simulink model "New_FOC_old0x2820x29"  (R2024b)
settings: Solver=FixedStepAuto  StartTime=0.0  StopTime=2.5  FixedStep=1e-6  MaxStep=1e-3
values from neighbouring files (symbols this model uses):
  Ki_d = (wn_d^2) / b_d    (= 228532.608696)    [FOC_Code.m]
  Ki_q = (wn_q^2) / b_q    (= 228532.608696)    [FOC_Code.m]
  Ki_s = (wn_s^2) / b_s    [FOC_Code.m]
  Kp_d = (2*zeta*wn_d - a_d) / b_d    (= 62.35)    [FOC_Code.m]
  Kp_q = (2*zeta*wn_q - a_q) / b_q    (= 62.35)    [FOC_Code.m]
  Kp_s = (2*zeta*wn_s - a_s) / b_s    [FOC_Code.m]
  lambda = 0.0884669    [FOC_Code.m]
  Ld = 5.75e-3    (= 0.00575)    [FOC_Code.m]
  Lq = 5.75e-3    (= 0.00575)    [FOC_Code.m]
  ma = 0.95    [FOC_Code.m]
  p = 3    [FOC_Code.m]
  T_max = 3.81    [FOC_Code.m]
  T_period = 1/fs    (= 0.0001)    [FOC_Code.m]
  Vdc = 311    [FOC_Code.m]
libraries: spsIGBTDiodeLib x12, simulink x9, spsCurrentMeasurementLib x6, spsVoltageMeasurementLib x6, spsStairGeneratorLib x3, spsDCVoltageSourceLib x2, spsPermanentMagnetSynchronousMachineLib x2, spsTriangleGeneratorLib x1, spspowerguiLib x1, sps_lib x1
settings Model: Creator=FSOS  LastModifiedBy=Habiba
settings SolverCC: ZeroCrossAlgorithm=Adaptive  AlgebraicLoopSolver=TrustRegion
settings DebuggingCC: IgnoredZcDiagnostic=none  ArithmeticOperatorsInVariantConditions=warning
settings SFSimCC: CustomCodeUndefinedFunction=UseInterfaceOnly
settings RTWCC: GPUComputeCapability=3.5

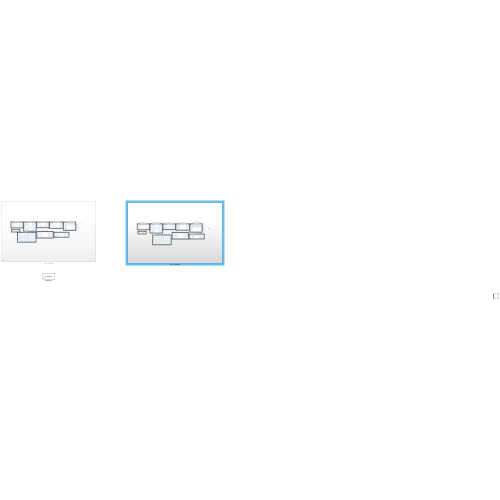
[thumbnail: Simulink's stored preview of the top-level diagram]
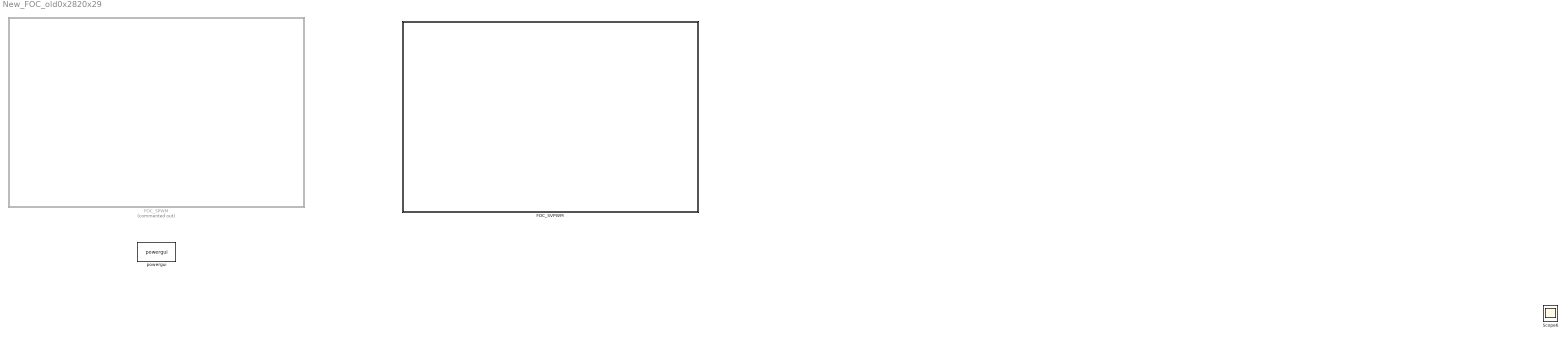
== system New_FOC_old0x2820x29 ==
  FOC_SPWM : Subsystem  Commented=on
  FOC_SVPWM : Subsystem
  Scope6 : Scope  NumInputPorts=3
  powergui : sps_lib/powergui  Priority=1  SimulationMode=Continuous  SampleTime=50e-6  frequency=60  Iterations=50  frequencyindice=0  Pbase=100e6  ErrMax=1e-4  UnitsV=kV  UnitsW=MW  buscounter=0  FunctionMessages=off  echomessages=off  EnableUseOfTLC=off  CurrentSourceSwitches=off  DisableSnubberDevices=off  DisableRonSwitches=off  DisableVfSwitches=off  DisplayEquations=off  AutomaticDiscreteSolvers=off  SolverType=Tustin/Backward Euler (TBE)  Interpol=off  ExternalGateDelay=off  methode=off  Ts=100  x0status=blocks  SPID=on  SwTol=0  HookPort=off  NonlinearTolerance=1e-4  nMaxIteration=100  ContinueOnMaxIteration=off  RestoreLinks=warning  ResistiveCurrentMeasurement=off  Frange=[0:2:500]  Ylog=off  Xlog=on  ShowGrid=off  save=off  variable=ZData  structure=0  ZoomFFT=off  StartTime=0.0  cycles=1  DisplayStyle=1  fundamental=60  FreqAxis=off  MaxFrequency=1000  frequencyindicesteady=1  RmsSteady=1  display=off

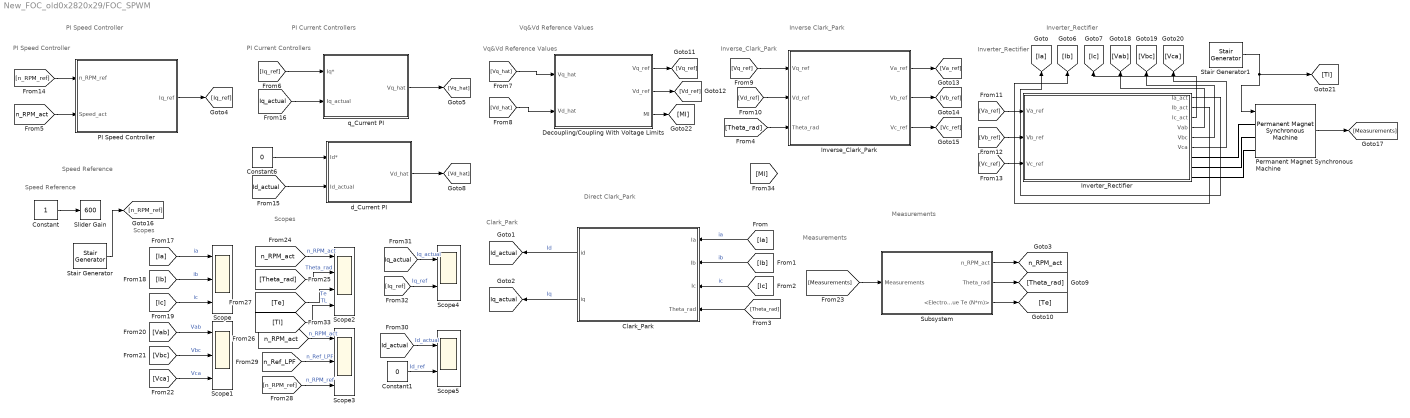
== system New_FOC_old0x2820x29/FOC_SPWM ==
  note: Scopes
  note: Measurements
  note: Speed Reference
  note: Inverter_Rectifier
  note: Clark_Park
  note: Inverse_Clark_Park
  note: Vq&Vd Reference Values
  note: PI Current Controllers
  note: PI Speed Controller
  note: PI Speed Controller
  note: PI Current Controllers
  note: Vq&Vd Reference Values
  note: Inverse Clark_Park
  note: Direct Clark_Park
  note: Inverter_Rectifier
  note: Speed Reference
  note: Measurements
  note: Scopes
  Clark_Park : Subsystem
  Constant : Constant
  Constant1 : Constant  Value=0
  Constant6 : Constant  Value=0
  Decoupling/Coupling With Voltage Limits : Subsystem
  Inverse_Clark_Park : Subsystem
  Inverter_Rectifier : Subsystem
  PI Speed Controller : Subsystem
  Permanent Magnet Synchronous Machine : spsPermanentMagnetSynchronousMachineLib/Permanent Magnet Synchronous Machine  NbPhases=3  FluxDistribution=Sinusoidal  RotorType=Round  MechanicalLoad=Torque Tm  PresetModel="01:  0.8 Nm 300 Vdc 3000 RPM - 0.8 Nm"  ShowDetailedParameters=on  MeasurementBus=off  Resistance=18.7  Inductance=8.5e-3  dqInductances=[0.006047 0.006683]  La=0.02682  MachineConstant=Flux linkage established by magnets (V.s)  Flux=0.1716  VoltageCst=62.2496  TorqueCst=0.5148  Flat=120  Mechanical=[2.26e-05 1.349e-05 2 0]  PolePairs=2  InitialConditions=[0,0, 0,0]  InitialConditions5ph=[0 0 0 0 0 0]  RefAngle=Aligned with phase A axis (original Park)  IterativeDiscreteModel=Trapezoidal non iterative  TsBlock=-1  TsPowergui=0
  Scope : Scope  NumInputPorts=3
  Scope1 : Scope  NumInputPorts=3
  Scope2 : Scope  NumInputPorts=4
  Scope3 : Scope  NumInputPorts=3
  Scope4 : Scope  NumInputPorts=2
  Scope5 : Scope  NumInputPorts=2
  Slider Gain : simulink/Math Operations/Slider Gain  gain=600  low=0  high=3000
  Stair Generator : spsStairGeneratorLib/Stair Generator  t=[0 .15 .3 .45 .7 .85 1 1.15 1.3]  e=[200 2000 500 3000 0 -1000 -2500 0 2500]  Ts=1e-5
  Stair Generator1 : spsStairGeneratorLib/Stair Generator  t=[0 1.3 1.45 1.6 1.75 1.9 2]  e=[0 1.5 2 2.8 2.5 .8 2.2]  Ts=0
  Subsystem : Subsystem
  d_Current PI : Subsystem
  q_Current PI : Subsystem
  tag scope: Id_actual=global, Iq_actual=global, n_RPM_act=global
  wires:
  Subsystem/2(Theta_rad) -> [Theta_rad]
  Constant6/1 -> d_Current PI/1(Id*)
  [Vd_ref] -> Inverse_Clark_Park/2(Vd_ref)
  [Vq_ref] -> Inverse_Clark_Park/1(Vq_ref)
  [n_RPM_ref] -> PI Speed Controller/1(n_RPM_ref)
  [Iq_actual] -> Scope4/1  "Iq_actual"
  [Id_actual] -> d_Current PI/2(Id_actual)
  Inverter_Rectifier/2(Ib_act) -> [Ib]
  [Ic] -> Clark_Park/3(Ic)  "ic"
  Inverse_Clark_Park/2(Vb_ref) -> [Vb_ref]
  Clark_Park/2(iq) -> [Iq_actual]  "Iq"
  [n_RPM_act] -> PI Speed Controller/2(Speed_act)
  [Ia] -> Scope/1  "ia"
  Clark_Park/1(id) -> [Id_actual]  "Id"
  [Iq_actual] -> q_Current PI/2(Iq_actual)
  [Iq_ref] -> Scope4/2  "Iq_ref"
  Decoupling/Coupling With Voltage Limits/2(Vd_ref) -> [Vd_ref]
  [Ib] -> Scope/2  "ib"
  Constant/1 -> Slider Gain/1
  [Ib] -> Clark_Park/2(Ib)  "ib"
  Inverter_Rectifier/5(Vbc) -> [Vbc]
  [Theta_rad] -> Inverse_Clark_Park/3(Theta_rad)
  [Id_actual] -> Scope5/1  "Id_actual"
  [Ia] -> Clark_Park/1(Ia)  "ia"
  [Theta_rad] -> Clark_Park/4(Theta_rad)
  [Measurements] -> Subsystem/1(Measurements)
  [Vq_hat] -> Decoupling/Coupling With Voltage Limits/1(Vq_hat)
  Decoupling/Coupling With Voltage Limits/1(Vq_ref) -> [Vq_ref]
  PI Speed Controller/1(Iq_ref) -> [Iq_ref]
  [Vca] -> Scope1/3  "Vca"
  d_Current PI/1(Vd_hat) -> [Vd_hat]
  [Vd_hat] -> Decoupling/Coupling With Voltage Limits/2(Vd_hat)
  [Va_ref] -> Inverter_Rectifier/1(Va_ref)
  Constant1/1 -> Scope5/2  "Id_ref"
  [Vc_ref] -> Inverter_Rectifier/3(Vc_ref)
  [n_RPM_act] -> Scope2/1  "n_RPM_act"
  Inverse_Clark_Park/3(Vc_ref) -> [Vc_ref]
  Inverter_Rectifier/6(Vca) -> [Vca]
  [Iq_ref] -> q_Current PI/1(Iq*)
  [Vab] -> Scope1/1  "Vab"
  q_Current PI/1(Vq_hat) -> [Vq_hat]
  Inverter_Rectifier/1(Ia_act) -> [Ia]
  [n_RPM_act] -> Scope3/1  "n_RPM_act"
  [Vb_ref] -> Inverter_Rectifier/2(Vb_ref)
  Subsystem/1(n_RPM_act) -> [n_RPM_act]
  [Theta_rad] -> Scope2/2  "Theta_rad"
  Inverter_Rectifier/4(Vab) -> [Vab]
  Inverter_Rectifier/3(Ic_act) -> [Ic]
  Inverse_Clark_Park/1(Va_ref) -> [Va_ref]
  [Te] -> Scope2/3  "Te"
  Subsystem/3(<Electromagnetic torque Te (N*m)>) -> [Te]
  [Ic] -> Scope/3  "ic"
  [Vbc] -> Scope1/2  "Vbc"
  Permanent Magnet Synchronous Machine/1 -> [Measurements]
  Stair Generator1/1 -> Permanent Magnet Synchronous Machine/1, [Tl]
  [Tl] -> Scope2/4  "TL"
  [n_Ref_LPF] -> Scope3/2  "n_Ref_LPF"
  [n_RPM_ref] -> Scope3/3  "n_RPM_ref"
  Decoupling/Coupling With Voltage Limits/3(MI) -> [MI]
  Stair Generator/1 -> [n_RPM_ref]
  connections:
  Permanent Magnet Synchronous Machine/LConn2 -- Inverter_Rectifier/RConn2
  Permanent Magnet Synchronous Machine/LConn1 -- Inverter_Rectifier/RConn1
  Permanent Magnet Synchronous Machine/LConn3 -- Inverter_Rectifier/RConn3

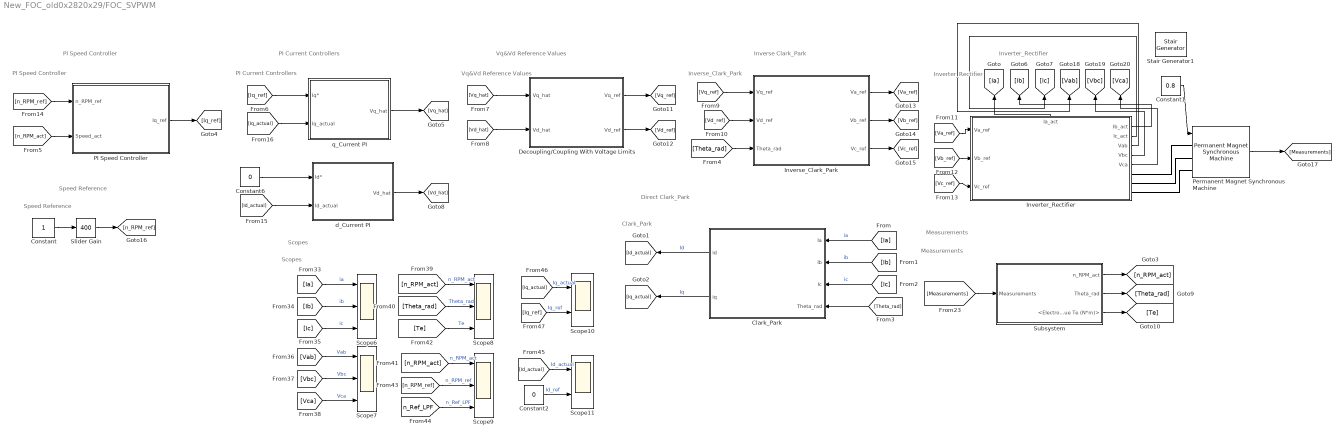
== system New_FOC_old0x2820x29/FOC_SVPWM ==
  note: Measurements
  note: Speed Reference
  note: Inverter_Rectifier
  note: Direct Clark_Park
  note: Inverse Clark_Park
  note: Vq&Vd Reference Values
  note: PI Current Controllers
  note: PI Speed Controller
  note: PI Speed Controller
  note: PI Current Controllers
  note: Vq&Vd Reference Values
  note: Inverse_Clark_Park
  note: Clark_Park
  note: Inverter_Rectifier
  note: Speed Reference
  note: Measurements
  note: Scopes
  note: Scopes
  Clark_Park : Subsystem
  Constant : Constant
  Constant1 : Constant  Value=0.8
  Constant2 : Constant  Value=0
  Constant6 : Constant  Value=0
  Decoupling/Coupling With Voltage Limits : Subsystem
  Inverse_Clark_Park : Subsystem
  Inverter_Rectifier : Subsystem
      settings: PortSchema="{\"entries\":[{\"content\":{\"sides\":[{\"content\":{\"connectorIds\":[\"In1\",\"In2\",\"In3\"]},\"type\":\"ConnectorPlacement.EquallySpacedRectSide\",\"uuid\":\"7414f413-f740-4713-9a5b-35e41764df99\"},{\"content\":{\"connectorIds\":[\"Out1\",\"Out2\",\"Out3\",\"Out4\",\"Out5\",\"RConn1\",\"RConn2\",\"RConn3\"],\"side\":\"RIGHT\"},\"type\":\"ConnectorPlacement.EquallySpacedRectSide\",\"uuid\":\"0ae7f1d1-4f19-4170-a25f-9376873eedc4\"},{\"content\":{\"connectorIds\":[\"Out6\"],\"side\":\"TOP\"},\"type\":\"ConnectorPlacement.EquallySpacedRectSide\",\"uuid\":\"dcf59177-a21c-40cb-b25d-eb83961f197b\"}]},\"type\":\"ConnectorPlacement.EquallySpacedConnector\",\"uuid\":\"0cdaba68-969f-44b0-8b53-9ca11596f6f2\"}],\"packageUris\":[\"http://schema.mathworks.com/mf0/Connector/R2020b\"],\"version\":\"1.0\"}"
  PI Speed Controller : Subsystem
  Permanent Magnet Synchronous Machine : spsPermanentMagnetSynchronousMachineLib/Permanent Magnet Synchronous Machine  NbPhases=3  FluxDistribution=Sinusoidal  RotorType=Round  MechanicalLoad=Torque Tm  PresetModel=No  ShowDetailedParameters=on  MeasurementBus=off  Resistance=2.9  Inductance=8.5e-3  dqInductances=[0.006047 0.006683]  La=5.75e-3  MachineConstant=Flux linkage established by magnets (V.s)  Flux=0.0884669  VoltageCst=48.1384  TorqueCst=0.3981  Flat=120  Mechanical=[0.405e-4 0.0314 3 0]  PolePairs=2  InitialConditions=[0,0, 0,0]  InitialConditions5ph=[0 0 0 0 0 0]  RefAngle=Aligned with phase A axis (original Park)  IterativeDiscreteModel=Trapezoidal non iterative  TsBlock=-1  TsPowergui=0
  Scope10 : Scope  NumInputPorts=2
  Scope11 : Scope  NumInputPorts=2
  Scope{6..9} (4 alike) : Scope  NumInputPorts=3
  Slider Gain : simulink/Math Operations/Slider Gain  gain=400  low=0  high=3000
  Stair Generator1 : spsStairGeneratorLib/Stair Generator  t=[0 1.3 1.45 1.6 1.75 1.9 2]  e=[0 1.5 2 2.8 2.5 .8 2.2]  Ts=0
  Subsystem : Subsystem
  d_Current PI : Subsystem
  q_Current PI : Subsystem
  wires:
  Permanent Magnet Synchronous Machine/1 -> [Measurements]
  Subsystem/3(<Electromagnetic torque Te (N*m)>) -> [Te]
  Inverse_Clark_Park/1(Va_ref) -> [Va_ref]
  Inverter_Rectifier/2(Ic_act) -> [Ic]
  Inverter_Rectifier/3(Vab) -> [Vab]
  Subsystem/1(n_RPM_act) -> [n_RPM_act]
  [Vb_ref] -> Inverter_Rectifier/2(Vb_ref)
  Inverter_Rectifier/6(Ia_act) -> [Ia]
  q_Current PI/1(Vq_hat) -> [Vq_hat]
  [Iq_ref] -> q_Current PI/1(Iq*)
  Inverter_Rectifier/5(Vca) -> [Vca]
  Inverse_Clark_Park/3(Vc_ref) -> [Vc_ref]
  [Vc_ref] -> Inverter_Rectifier/3(Vc_ref)
  [Va_ref] -> Inverter_Rectifier/1(Va_ref)
  [Vd_hat] -> Decoupling/Coupling With Voltage Limits/2(Vd_hat)
  d_Current PI/1(Vd_hat) -> [Vd_hat]
  PI Speed Controller/1(Iq_ref) -> [Iq_ref]
  Decoupling/Coupling With Voltage Limits/1(Vq_ref) -> [Vq_ref]
  [Vq_hat] -> Decoupling/Coupling With Voltage Limits/1(Vq_hat)
  [Measurements] -> Subsystem/1(Measurements)
  [Theta_rad] -> Clark_Park/4(Theta_rad)
  [Ia] -> Clark_Park/1(Ia)  "ia"
  [Theta_rad] -> Inverse_Clark_Park/3(Theta_rad)
  Inverter_Rectifier/4(Vbc) -> [Vbc]
  [Ib] -> Clark_Park/2(Ib)  "ib"
  Constant/1 -> Slider Gain/1
  Decoupling/Coupling With Voltage Limits/2(Vd_ref) -> [Vd_ref]
  [Iq_actual] -> q_Current PI/2(Iq_actual)
  Clark_Park/1(id) -> [Id_actual]  "Id"
  [n_RPM_act] -> PI Speed Controller/2(Speed_act)
  Clark_Park/2(iq) -> [Iq_actual]  "Iq"
  Inverse_Clark_Park/2(Vb_ref) -> [Vb_ref]
  [Ic] -> Clark_Park/3(Ic)  "ic"
  Inverter_Rectifier/1(Ib_act) -> [Ib]
  [Id_actual] -> d_Current PI/2(Id_actual)
  [n_RPM_ref] -> PI Speed Controller/1(n_RPM_ref)
  [Vq_ref] -> Inverse_Clark_Park/1(Vq_ref)
  [Vd_ref] -> Inverse_Clark_Park/2(Vd_ref)
  Constant6/1 -> d_Current PI/1(Id*)
  Subsystem/2(Theta_rad) -> [Theta_rad]
  [n_RPM_act] -> Scope9/1  "n_RPM_act"
  [n_RPM_act] -> Scope8/1  "n_RPM_act"
  [Theta_rad] -> Scope8/2  "Theta_rad"
  [Vca] -> Scope7/3  "Vca"
  [Ia] -> Scope6/1  "ia"
  [n_Ref_LPF] -> Scope9/3  "n_Ref_LPF"
  [Id_actual] -> Scope11/1  "Id_actual"
  Constant2/1 -> Scope11/2  "Id_ref"
  [Iq_actual] -> Scope10/1  "Iq_actual"
  [Vbc] -> Scope7/2  "Vbc"
  [Te] -> Scope8/3  "Te"
  [Iq_ref] -> Scope10/2  "Iq_ref"
  [Vab] -> Scope7/1  "Vab"
  [Ic] -> Scope6/3  "ic"
  [n_RPM_ref] -> Scope9/2  "n_RPM_ref"
  [Ib] -> Scope6/2  "ib"
  Constant1/1 -> Permanent Magnet Synchronous Machine/1
  Slider Gain/1 -> [n_RPM_ref]
  connections:
  Permanent Magnet Synchronous Machine/LConn3 -- Inverter_Rectifier/RConn3
  Permanent Magnet Synchronous Machine/LConn1 -- Inverter_Rectifier/RConn1
  Permanent Magnet Synchronous Machine/LConn2 -- Inverter_Rectifier/RConn2

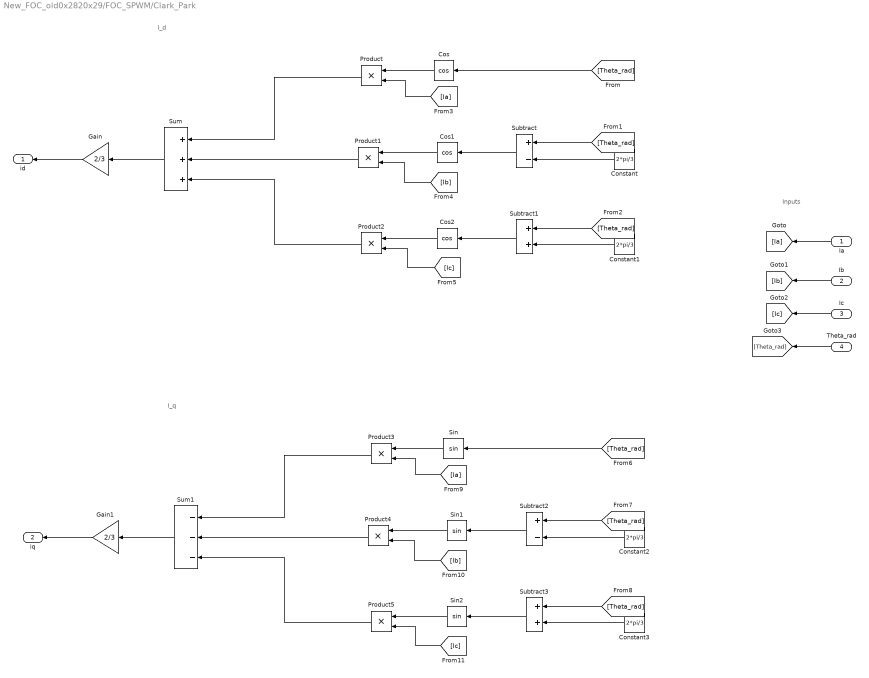
== system New_FOC_old0x2820x29/FOC_SPWM/Clark_Park ==
  note: Inputs
  note: I_d
  note: I_q
  Ia : Inport
  Ib : Inport  Port=2
  Ic : Inport  Port=3
  Theta_rad : Inport  Port=4
  Constant{,1..3} (4 alike) : Constant  Value=2*pi/3
  Cos : Trigonometry  Operator=cos
  Cos1 : Trigonometry  Operator=cos
  Cos2 : Trigonometry  Operator=cos
  Gain : Gain  Gain=2/3
  Gain1 : Gain  Gain=2/3
  Product{,1..5} (6 alike) : Product
  Sin : Trigonometry
  Sin1 : Trigonometry
  Sin2 : Trigonometry
  Subtract : Sum  Inputs=+-
  Subtract1 : Sum
  Subtract2 : Sum  Inputs=+-
  Subtract3 : Sum
  Sum : Sum  Inputs=+++
  Sum1 : Sum  Inputs=---
  id : Outport
  iq : Outport  Port=2
  wires:
  Ia/1 -> [Ia]
  Ib/1 -> [Ib]
  Ic/1 -> [Ic]
  Theta_rad/1 -> [Theta_rad]
  Cos/1 -> Product/1
  Cos1/1 -> Product1/1
  Cos2/1 -> Product2/1
  [Theta_rad] -> Cos/1
  Subtract/1 -> Cos1/1
  [Theta_rad] -> Subtract/1
  Constant/1 -> Subtract/2
  Constant1/1 -> Subtract1/2
  [Theta_rad] -> Subtract1/1
  Subtract1/1 -> Cos2/1
  [Ia] -> Product/2
  [Ib] -> Product1/2
  [Ic] -> Product2/2
  Product1/1 -> Sum/2
  Product/1 -> Sum/1
  Product2/1 -> Sum/3
  Sum/1 -> Gain/1
  Gain/1 -> id/1
  Gain1/1 -> iq/1
  Sum1/1 -> Gain1/1
  Product5/1 -> Sum1/3
  Product3/1 -> Sum1/1
  Product4/1 -> Sum1/2
  [Ic] -> Product5/2
  [Ib] -> Product4/2
  [Ia] -> Product3/2
  Subtract3/1 -> Sin2/1
  [Theta_rad] -> Subtract3/1
  Constant3/1 -> Subtract3/2
  Constant2/1 -> Subtract2/2
  [Theta_rad] -> Subtract2/1
  Subtract2/1 -> Sin1/1
  [Theta_rad] -> Sin/1
  Sin2/1 -> Product5/1
  Sin1/1 -> Product4/1
  Sin/1 -> Product3/1

== system New_FOC_old0x2820x29/FOC_SPWM/Decoupling//Coupling With Voltage Limits ==
  note: MI_Calculations
  Vq_hat : Inport
  Vd_hat : Inport  Port=2
  Decoupling/Coupling : Subsystem
  MI_Calculations : Subsystem
  Voltage Limited : Subsystem
  Vq_ref : Outport
  Vd_ref : Outport  Port=2
  MI : Outport  Port=3
  wires:
  Decoupling/Coupling/1(Vq) -> Voltage Limited/1(Vq)
  Decoupling/Coupling/2(Vd) -> Voltage Limited/2(Vd)
  Vq_hat/1 -> Decoupling/Coupling/1(Vq_hat)
  Voltage Limited/1(Vq_ref) -> MI_Calculations/1(Vq_ref), Vq_ref/1
  Vd_hat/1 -> Decoupling/Coupling/2(Vd_hat)
  MI_Calculations/1(MI) -> MI/1
  Voltage Limited/2(Vd_ref) -> MI_Calculations/2(Vd_ref), Vd_ref/1

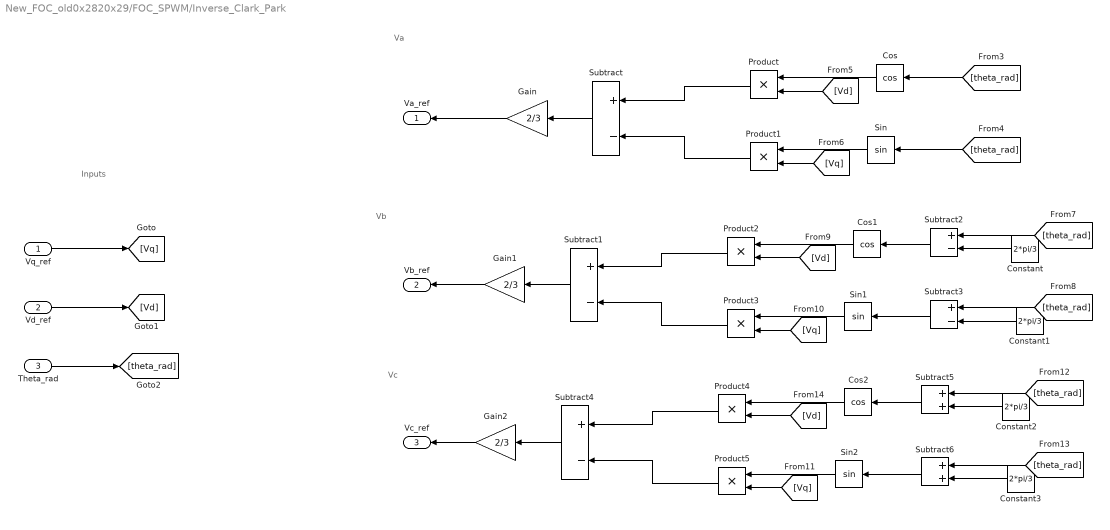
== system New_FOC_old0x2820x29/FOC_SPWM/Inverse_Clark_Park ==
  note: Vc
  note: Vb
  note: Va
  note: Inputs
  Vq_ref : Inport
  Vd_ref : Inport  Port=2
  Theta_rad : Inport  Port=3
  Constant{,1..3} (4 alike) : Constant  Value=2*pi/3
  Cos : Trigonometry  Operator=cos
  Cos1 : Trigonometry  Operator=cos
  Cos2 : Trigonometry  Operator=cos
  Gain : Gain  Gain=2/3
  Gain1 : Gain  Gain=2/3
  Gain2 : Gain  Gain=2/3
  Product{,1..5} (6 alike) : Product
  Sin : Trigonometry
  Sin1 : Trigonometry
  Sin2 : Trigonometry
  Subtract{,1..4} (5 alike) : Sum  Inputs=+-
  Subtract5 : Sum
  Subtract6 : Sum
  Va_ref : Outport
  Vb_ref : Outport  Port=2
  Vc_ref : Outport  Port=3
  wires:
  Vq_ref/1 -> [Vq]
  Vd_ref/1 -> [Vd]
  Theta_rad/1 -> [theta_rad]
  [theta_rad] -> Cos/1
  [theta_rad] -> Sin/1
  Cos/1 -> Product/1
  Sin/1 -> Product1/1
  [Vd] -> Product/2
  [Vq] -> Product1/2
  Product/1 -> Subtract/1
  Product1/1 -> Subtract/2
  Subtract/1 -> Gain/1
  Gain/1 -> Va_ref/1
  Subtract1/1 -> Gain1/1
  Product3/1 -> Subtract1/2
  Product2/1 -> Subtract1/1
  [Vq] -> Product3/2
  [Vd] -> Product2/2
  Sin1/1 -> Product3/1
  Cos1/1 -> Product2/1
  Subtract2/1 -> Cos1/1
  [theta_rad] -> Subtract2/1
  Subtract3/1 -> Sin1/1
  [theta_rad] -> Subtract3/1
  Constant/1 -> Subtract2/2
  Constant1/1 -> Subtract3/2
  Gain1/1 -> Vb_ref/1
  Gain2/1 -> Vc_ref/1
  Constant3/1 -> Subtract6/2
  Constant2/1 -> Subtract5/2
  [theta_rad] -> Subtract6/1
  Subtract6/1 -> Sin2/1
  [theta_rad] -> Subtract5/1
  Subtract5/1 -> Cos2/1
  Cos2/1 -> Product4/1
  Sin2/1 -> Product5/1
  [Vd] -> Product4/2
  [Vq] -> Product5/2
  Product4/1 -> Subtract4/1
  Product5/1 -> Subtract4/2
  Subtract4/1 -> Gain2/1

== system New_FOC_old0x2820x29/FOC_SPWM/Inverter_Rectifier ==
  Va_ref : Inport
  Vb_ref : Inport  Port=2
  Vc_ref : Inport  Port=3
  Current Measurement : spsCurrentMeasurementLib/Current Measurement  PhasorSimulation=off  OutputType=Complex  PSBequivalent=0
  Current Measurement1 : spsCurrentMeasurementLib/Current Measurement  PhasorSimulation=off  OutputType=Complex  PSBequivalent=0
  Current Measurement2 : spsCurrentMeasurementLib/Current Measurement  PhasorSimulation=off  OutputType=Complex  PSBequivalent=0
  Inverter_SPWM : Subsystem
  Voltage Measurement : spsVoltageMeasurementLib/Voltage Measurement  PhasorSimulation=off  OutputType=Complex  PSBequivalent=0
  Voltage Measurement1 : spsVoltageMeasurementLib/Voltage Measurement  PhasorSimulation=off  OutputType=Complex  PSBequivalent=0
  Voltage Measurement2 : spsVoltageMeasurementLib/Voltage Measurement  PhasorSimulation=off  OutputType=Complex  PSBequivalent=0
  Va_act : PMIOPort  Side=Right
  Vb_act : PMIOPort  Port=2  Side=Right
  Vc_act : PMIOPort  Port=3  Side=Right
  Ia_act : Outport
  Ib_act : Outport  Port=2
  Ic_act : Outport  Port=3
  Vab : Outport  Port=4
  Vbc : Outport  Port=5
  Vca : Outport  Port=6
  wires:
  Current Measurement/1 -> Ia_act/1
  Vc_ref/1 -> Inverter_SPWM/3(Vc_ref)
  Current Measurement2/1 -> Ic_act/1
  Current Measurement1/1 -> Ib_act/1
  Vb_ref/1 -> Inverter_SPWM/2(Vb_ref)
  Va_ref/1 -> Inverter_SPWM/1(Va_ref)
  Voltage Measurement/1 -> Vab/1
  Voltage Measurement1/1 -> Vbc/1
  Voltage Measurement2/1 -> Vca/1
  connections:
  Current Measurement/RConn1 -- Va_act/RConn1
  Current Measurement1/RConn1 -- Vb_act/RConn1
  Current Measurement/LConn1 -- Inverter_SPWM/RConn1 -- Voltage Measurement2/LConn2 -- Voltage Measurement/LConn1
  Inverter_SPWM/RConn3 -- Voltage Measurement1/LConn2 -- Current Measurement2/LConn1 -- Voltage Measurement2/LConn1
  Inverter_SPWM/RConn2 -- Voltage Measurement/LConn2 -- Current Measurement1/LConn1 -- Voltage Measurement1/LConn1
  Current Measurement2/RConn1 -- Vc_act/RConn1

== system New_FOC_old0x2820x29/FOC_SPWM/PI Speed Controller ==
  note: في لوك لتحويل للrad/s
  note: Subsystem2
  n_RPM_ref : Inport
  Speed_act : Inport  Port=2
  Abs : Abs  SaturateOnIntegerOverflow=off
  Abs1 : Abs  SaturateOnIntegerOverflow=off
  Compare To Constant : simulink/Logic and Bit Operations/Compare To Constant  relop=<=  const=0.0001  OutDataTypeStr=boolean
  For stop integral in the starting : Relay  OnSwitchValue=100  OffSwitchValue=-100
  Gain : Gain  Gain=Kp_s
  Gain1 : Gain  Gain=Ki_s
  Integrator1 : Integrator
  Iq_Max : Saturate  UpperLimit=T_max*2/(3*p*lambda)  LowerLimit=-(2*T_max) / (3*p*lambda)
  LPF : TransferFcn  Denominator=[1/100 1]
  Product : Product  Inputs=3
  Sum : Sum  Inputs=|+-
  Sum3 : Sum  Inputs=|++
  Sum4 : Sum  Inputs=|-+
  Iq_ref : Outport
  tag scope: n_Ref_LPF=global
  wires:
  Speed_act/1 -> Abs1/1, Sum/2
  Iq_Max/1 -> Iq_ref/1, Sum4/1
  LPF/1 -> [n_Ref_LPF], Sum/1
  Gain1/1 -> Product/2
  Sum3/1 -> Sum4/2, Iq_Max/1
  Gain/1 -> Sum3/1
  Abs1/1 -> For stop integral in the starting/1
  Product/1 -> Integrator1/1
  For stop integral in the starting/1 -> Product/3
  Integrator1/1 -> Sum3/2
  Sum4/1 -> Abs/1
  Abs/1 -> Compare To Constant/1
  Compare To Constant/1 -> Product/1
  n_RPM_ref/1 -> LPF/1
  Sum/1 -> Gain1/1, Gain/1

== system New_FOC_old0x2820x29/FOC_SPWM/Subsystem ==
  Measurements : Inport
  0-2pi : Math  Operator=rem  SignedPower=on
  Bus Selector : BusSelector  OutputSignals=Rotor speed wm (rad/s),Rotor angle thetam (rad),Electromagnetic torque Te (N*m)
  Constant7 : Constant  Value=2*pi
  Gain2 : Gain  Gain=30/pi
  mech to elec1 : Gain  Gain=p
  n_RPM_act : Outport
  Theta_rad : Outport  Port=2
  <Electromagnetic torque Te (N*m)> : Outport  Port=3
  wires:
  Constant7/1 -> 0-2pi/2
  Measurements/1 -> Bus Selector/1
  Gain2/1 -> n_RPM_act/1
  Bus Selector/1 -> Gain2/1  "<Rotor speed wm (rad/s)>"
  Bus Selector/2 -> mech to elec1/1  "<Rotor angle thetam (rad)>"
  Bus Selector/3 -> <Electromagnetic torque Te (N*m)>/1  "<Electromagnetic torque Te (N*m)>"
  0-2pi/1 -> Theta_rad/1
  mech to elec1/1 -> 0-2pi/1

== system New_FOC_old0x2820x29/FOC_SPWM/d_Current PI ==
  Id* : Inport
  Id_actual : Inport  Port=2
  Gain : Gain  Gain=Kp_d
  Gain1 : Gain  Gain=Ki_d
  Integrator : Integrator
  Product : Product
  Sum : Sum  Inputs=|+-
  Sum1 : Sum  Inputs=|++
  Vd_hat : Outport
  wires:
  Sum1/1 -> Vd_hat/1
  Gain1/1 -> Product/1
  Gain/1 -> Sum1/1
  Sum/1 -> Gain/1, Gain1/1
  Id_actual/1 -> Sum/2
  Id*/1 -> Sum/1
  [Stop_d] -> Product/2  "act as anti wind-up"
  Product/1 -> Integrator/1
  Integrator/1 -> Sum1/2

== system New_FOC_old0x2820x29/FOC_SPWM/q_Current PI ==
  Iq* : Inport
  Iq_actual : Inport  Port=2
  Gain : Gain  Gain=Kp_q
  Gain1 : Gain  Gain=Ki_q
  Integrator : Integrator
  Product : Product
  Sum : Sum  Inputs=|+-
  Sum1 : Sum  Inputs=|++
  Vq_hat : Outport
  wires:
  Iq*/1 -> Sum/1
  Iq_actual/1 -> Sum/2
  Sum/1 -> Gain1/1, Gain/1
  Gain/1 -> Sum1/1
  Gain1/1 -> Product/1
  Sum1/1 -> Vq_hat/1
  [Stop_q] -> Product/2  "act as anti wind-up"
  Integrator/1 -> Sum1/2
  Product/1 -> Integrator/1

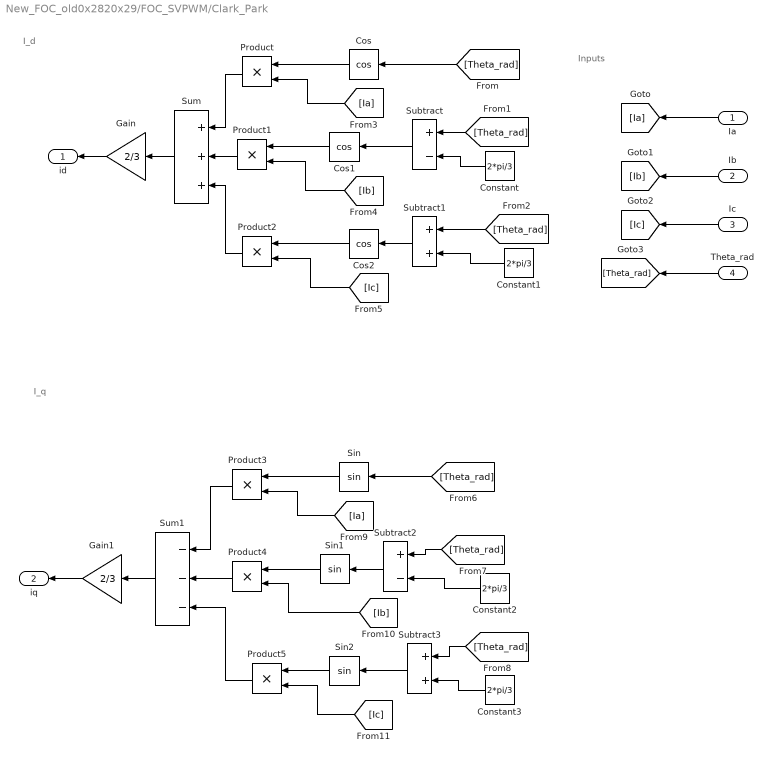
== system New_FOC_old0x2820x29/FOC_SVPWM/Clark_Park ==
  note: I_q
  note: I_d
  note: Inputs
  Ia : Inport
  Ib : Inport  Port=2
  Ic : Inport  Port=3
  Theta_rad : Inport  Port=4
  Constant{,1..3} (4 alike) : Constant  Value=2*pi/3
  Cos : Trigonometry  Operator=cos
  Cos1 : Trigonometry  Operator=cos
  Cos2 : Trigonometry  Operator=cos
  Gain : Gain  Gain=2/3
  Gain1 : Gain  Gain=2/3
  Product{,1..5} (6 alike) : Product
  Sin : Trigonometry
  Sin1 : Trigonometry
  Sin2 : Trigonometry
  Subtract : Sum  Inputs=+-
  Subtract1 : Sum
  Subtract2 : Sum  Inputs=+-
  Subtract3 : Sum
  Sum : Sum  Inputs=+++
  Sum1 : Sum  Inputs=---
  id : Outport
  iq : Outport  Port=2
  wires:
  Sin/1 -> Product3/1
  Sin1/1 -> Product4/1
  Sin2/1 -> Product5/1
  [Theta_rad] -> Sin/1
  Subtract2/1 -> Sin1/1
  [Theta_rad] -> Subtract2/1
  Constant2/1 -> Subtract2/2
  Constant3/1 -> Subtract3/2
  [Theta_rad] -> Subtract3/1
  Subtract3/1 -> Sin2/1
  [Ia] -> Product3/2
  [Ib] -> Product4/2
  [Ic] -> Product5/2
  Product4/1 -> Sum1/2
  Product3/1 -> Sum1/1
  Product5/1 -> Sum1/3
  Sum1/1 -> Gain1/1
  Gain1/1 -> iq/1
  Gain/1 -> id/1
  Sum/1 -> Gain/1
  Product2/1 -> Sum/3
  Product/1 -> Sum/1
  Product1/1 -> Sum/2
  [Ic] -> Product2/2
  [Ib] -> Product1/2
  [Ia] -> Product/2
  Subtract1/1 -> Cos2/1
  [Theta_rad] -> Subtract1/1
  Constant1/1 -> Subtract1/2
  Constant/1 -> Subtract/2
  [Theta_rad] -> Subtract/1
  Subtract/1 -> Cos1/1
  [Theta_rad] -> Cos/1
  Cos2/1 -> Product2/1
  Cos1/1 -> Product1/1
  Cos/1 -> Product/1
  Theta_rad/1 -> [Theta_rad]
  Ic/1 -> [Ic]
  Ib/1 -> [Ib]
  Ia/1 -> [Ia]

== system New_FOC_old0x2820x29/FOC_SVPWM/Decoupling//Coupling With Voltage Limits ==
  Vq_hat : Inport
  Vd_hat : Inport  Port=2
  Decoupling/Coupling : Subsystem
  Voltage Limited : Subsystem
  Vq_ref : Outport
  Vd_ref : Outport  Port=2
  wires:
  Voltage Limited/2(Vd*) -> Vd_ref/1
  Vq_hat/1 -> Decoupling/Coupling/1(Vq_hat)
  Vd_hat/1 -> Decoupling/Coupling/2(Vd_hat)
  Voltage Limited/1(Vq*) -> Vq_ref/1
  Decoupling/Coupling/2(Vd) -> Voltage Limited/2(Vd)
  Decoupling/Coupling/1(Vq) -> Voltage Limited/1(Vq)

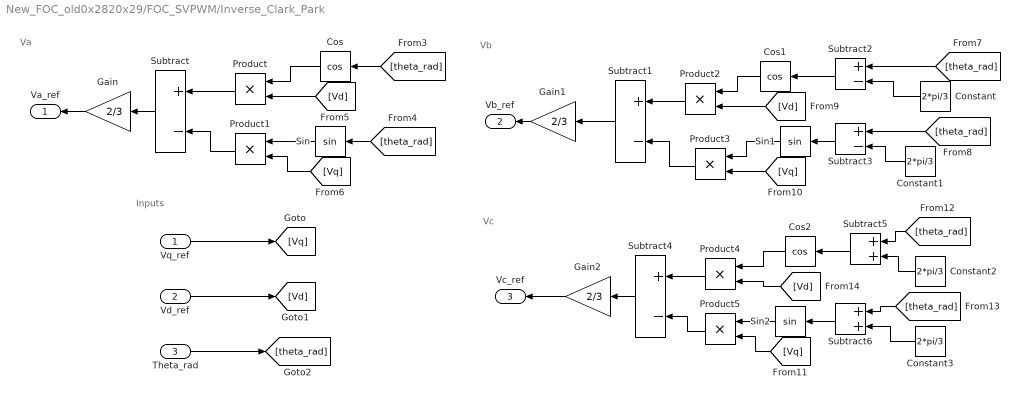
== system New_FOC_old0x2820x29/FOC_SVPWM/Inverse_Clark_Park ==
  note: Inputs
  note: Va
  note: Vb
  note: Vc
  Vq_ref : Inport
  Vd_ref : Inport  Port=2
  Theta_rad : Inport  Port=3
  Constant{,1..3} (4 alike) : Constant  Value=2*pi/3
  Cos : Trigonometry  Operator=cos
  Cos1 : Trigonometry  Operator=cos
  Cos2 : Trigonometry  Operator=cos
  Gain : Gain  Gain=2/3
  Gain1 : Gain  Gain=2/3
  Gain2 : Gain  Gain=2/3
  Product{,1..5} (6 alike) : Product
  Sin : Trigonometry
  Sin1 : Trigonometry
  Sin2 : Trigonometry
  Subtract{,1..4} (5 alike) : Sum  Inputs=+-
  Subtract5 : Sum
  Subtract6 : Sum
  Va_ref : Outport
  Vb_ref : Outport  Port=2
  Vc_ref : Outport  Port=3
  wires:
  Subtract4/1 -> Gain2/1
  Product5/1 -> Subtract4/2
  Product4/1 -> Subtract4/1
  [Vq] -> Product5/2
  [Vd] -> Product4/2
  Sin2/1 -> Product5/1
  Cos2/1 -> Product4/1
  Subtract5/1 -> Cos2/1
  [theta_rad] -> Subtract5/1
  Subtract6/1 -> Sin2/1
  [theta_rad] -> Subtract6/1
  Constant2/1 -> Subtract5/2
  Constant3/1 -> Subtract6/2
  Gain2/1 -> Vc_ref/1
  Gain1/1 -> Vb_ref/1
  Constant1/1 -> Subtract3/2
  Constant/1 -> Subtract2/2
  [theta_rad] -> Subtract3/1
  Subtract3/1 -> Sin1/1
  [theta_rad] -> Subtract2/1
  Subtract2/1 -> Cos1/1
  Cos1/1 -> Product2/1
  Sin1/1 -> Product3/1
  [Vd] -> Product2/2
  [Vq] -> Product3/2
  Product2/1 -> Subtract1/1
  Product3/1 -> Subtract1/2
  Subtract1/1 -> Gain1/1
  Gain/1 -> Va_ref/1
  Subtract/1 -> Gain/1
  Product1/1 -> Subtract/2
  Product/1 -> Subtract/1
  [Vq] -> Product1/2
  [Vd] -> Product/2
  Sin/1 -> Product1/1
  Cos/1 -> Product/1
  [theta_rad] -> Sin/1
  [theta_rad] -> Cos/1
  Theta_rad/1 -> [theta_rad]
  Vd_ref/1 -> [Vd]
  Vq_ref/1 -> [Vq]

== system New_FOC_old0x2820x29/FOC_SVPWM/Inverter_Rectifier ==
  Va_ref : Inport
  Vb_ref : Inport  Port=2
  Vc_ref : Inport  Port=3
  Current Measurement : spsCurrentMeasurementLib/Current Measurement  PhasorSimulation=off  OutputType=Complex  PSBequivalent=0
  Current Measurement1 : spsCurrentMeasurementLib/Current Measurement  PhasorSimulation=off  OutputType=Complex  PSBequivalent=0
  Current Measurement2 : spsCurrentMeasurementLib/Current Measurement  PhasorSimulation=off  OutputType=Complex  PSBequivalent=0
  Inverter_Three Phase SVPWM Mode : Subsystem
  Voltage Measurement : spsVoltageMeasurementLib/Voltage Measurement  PhasorSimulation=off  OutputType=Complex  PSBequivalent=0
  Voltage Measurement1 : spsVoltageMeasurementLib/Voltage Measurement  PhasorSimulation=off  OutputType=Complex  PSBequivalent=0
  Voltage Measurement2 : spsVoltageMeasurementLib/Voltage Measurement  PhasorSimulation=off  OutputType=Complex  PSBequivalent=0
  Va_act : PMIOPort  Side=Right
  Vb_act : PMIOPort  Port=2  Side=Right
  Vc_act : PMIOPort  Port=3  Side=Right
  Ib_act : Outport
  Ic_act : Outport  Port=2
  Vab : Outport  Port=3
  Vbc : Outport  Port=4
  Vca : Outport  Port=5
  Ia_act : Outport  Port=6
  wires:
  Voltage Measurement2/1 -> Vca/1
  Va_ref/1 -> Inverter_Three Phase SVPWM Mode/1(Va_ref)
  Vb_ref/1 -> Inverter_Three Phase SVPWM Mode/2(Vb_ref)
  Vc_ref/1 -> Inverter_Three Phase SVPWM Mode/3(Vc_ref)
  Current Measurement/1 -> Ia_act/1
  Current Measurement1/1 -> Ib_act/1
  Voltage Measurement/1 -> Vab/1
  Current Measurement2/1 -> Ic_act/1
  Voltage Measurement1/1 -> Vbc/1
  connections:
  Voltage Measurement2/LConn2 -- Inverter_Three Phase SVPWM Mode/RConn1 -- Voltage Measurement/LConn1 -- Current Measurement/LConn1
  Current Measurement/RConn1 -- Va_act/RConn1
  Inverter_Three Phase SVPWM Mode/RConn2 -- Voltage Measurement/LConn2 -- Current Measurement1/LConn1 -- Voltage Measurement1/LConn1
  Inverter_Three Phase SVPWM Mode/RConn3 -- Voltage Measurement2/LConn1 -- Voltage Measurement1/LConn2 -- Current Measurement2/LConn1
  Current Measurement1/RConn1 -- Vb_act/RConn1
  Current Measurement2/RConn1 -- Vc_act/RConn1

== system New_FOC_old0x2820x29/FOC_SVPWM/PI Speed Controller ==
  note: Subsystem2
  n_RPM_ref : Inport
  Speed_act : Inport  Port=2
  Abs : Abs  SaturateOnIntegerOverflow=off
  Abs1 : Abs  SaturateOnIntegerOverflow=off
  Compare To Constant : simulink/Logic and Bit Operations/Compare To Constant  relop=<=  const=0.0001  OutDataTypeStr=boolean
  For stop integral in the starting : Relay  OnSwitchValue=100  OffSwitchValue=-100
  Gain : Gain  Gain=Kp_s
  Gain1 : Gain  Gain=Ki_s
  Gain2 : Gain  Gain=pi/30
  Integrator1 : Integrator
  Iq_Max : Saturate  UpperLimit=T_max*2/(3*p*lambda)  LowerLimit=-(2*T_max) / (3*p*lambda)
  LPF : TransferFcn  Denominator=[1/100 1]
  Product : Product  Inputs=3
  Sum : Sum  Inputs=|+-
  Sum3 : Sum  Inputs=|++
  Sum4 : Sum  Inputs=|-+
  Iq_ref : Outport
  tag scope: n_Ref_LPF=global
  wires:
  Gain2/1 -> Gain/1, Gain1/1
  n_RPM_ref/1 -> LPF/1
  Compare To Constant/1 -> Product/1
  Abs/1 -> Compare To Constant/1
  Sum4/1 -> Abs/1
  Integrator1/1 -> Sum3/2
  For stop integral in the starting/1 -> Product/3
  Sum/1 -> Gain2/1
  Product/1 -> Integrator1/1
  Abs1/1 -> For stop integral in the starting/1
  Gain/1 -> Sum3/1
  Sum3/1 -> Sum4/2, Iq_Max/1
  Gain1/1 -> Product/2
  LPF/1 -> Sum/1, [n_Ref_LPF]
  Iq_Max/1 -> Sum4/1, Iq_ref/1
  Speed_act/1 -> Abs1/1, Sum/2

== system New_FOC_old0x2820x29/FOC_SVPWM/Subsystem ==
  Measurements : Inport
  0-2pi : Math  Operator=rem  SignedPower=on
  Bus Selector : BusSelector  OutputSignals=Rotor speed wm (rad/s),Rotor angle thetam (rad),Electromagnetic torque Te (N*m)
  Constant7 : Constant  Value=2*pi
  Gain2 : Gain  Gain=30/pi
  mech to elec1 : Gain  Gain=p
  n_RPM_act : Outport
  Theta_rad : Outport  Port=2
  <Electromagnetic torque Te (N*m)> : Outport  Port=3
  wires:
  Measurements/1 -> Bus Selector/1
  Bus Selector/2 -> mech to elec1/1  "<Rotor angle thetam (rad)>"
  Bus Selector/1 -> Gain2/1  "<Rotor speed wm (rad/s)>"
  Constant7/1 -> 0-2pi/2
  Bus Selector/3 -> <Electromagnetic torque Te (N*m)>/1  "<Electromagnetic torque Te (N*m)>"
  Gain2/1 -> n_RPM_act/1
  mech to elec1/1 -> 0-2pi/1
  0-2pi/1 -> Theta_rad/1

== system New_FOC_old0x2820x29/FOC_SVPWM/d_Current PI ==
  Id* : Inport
  Id_actual : Inport  Port=2
  Gain : Gain  Gain=Kp_d
  Gain1 : Gain  Gain=Ki_d
  Integrator : Integrator
  Product : Product
  Sum : Sum  Inputs=|+-
  Sum1 : Sum  Inputs=|++
  Vd_hat : Outport
  wires:
  Integrator/1 -> Sum1/2
  Product/1 -> Integrator/1
  [Stop_d] -> Product/2  "act as anti wind-up"
  Id*/1 -> Sum/1
  Id_actual/1 -> Sum/2
  Sum/1 -> Gain/1, Gain1/1
  Gain/1 -> Sum1/1
  Gain1/1 -> Product/1
  Sum1/1 -> Vd_hat/1

== system New_FOC_old0x2820x29/FOC_SVPWM/q_Current PI ==
  Iq* : Inport
  Iq_actual : Inport  Port=2
  Gain : Gain  Gain=Kp_q
  Gain1 : Gain  Gain=Ki_q
  Integrator : Integrator
  Product : Product
  Sum : Sum  Inputs=|+-
  Sum1 : Sum  Inputs=|++
  Vq_hat : Outport
  wires:
  Product/1 -> Integrator/1
  Integrator/1 -> Sum1/2
  [Stop_q] -> Product/2  "act as anti wind-up"
  Sum1/1 -> Vq_hat/1
  Gain1/1 -> Product/1
  Gain/1 -> Sum1/1
  Sum/1 -> Gain1/1, Gain/1
  Iq_actual/1 -> Sum/2
  Iq*/1 -> Sum/1

== system New_FOC_old0x2820x29/FOC_SPWM/Decoupling//Coupling With Voltage Limits/Decoupling//Coupling ==
  Vq_hat : Inport
  Vd_hat : Inport  Port=2
  Constant1 : Constant  Value=lambda
  Constant3 : Constant  Value=Ld
  Constant5 : Constant  Value=Lq
  Gain : Gain  Gain=pi/30
  Gain1 : Gain  Gain=pi/30
  Gain2 : Gain  Gain=pi/30
  Product3 : Product
  Product4 : Product  Inputs=3
  Product5 : Product  Inputs=3
  Sum1 : Sum  Inputs=|+-
  Sum2 : Sum  Inputs=+++
  Vq : Outport
  Vd : Outport  Port=2
  wires:
  Product3/1 -> Sum2/3
  Constant5/1 -> Product5/2
  [Iq_actual] -> Product5/3
  Constant1/1 -> Product3/2
  Sum2/1 -> Vq/1
  Product5/1 -> Sum1/2
  Gain2/1 -> Product5/1
  [Id_actual] -> Product4/3
  Gain1/1 -> Product3/1
  Gain/1 -> Product4/1
  Constant3/1 -> Product4/2
  Product4/1 -> Sum2/1
  Vd_hat/1 -> Sum1/1
  Sum1/1 -> Vd/1
  Vq_hat/1 -> Sum2/2
  [n_RPM_act] -> Gain/1
  [n_RPM_act] -> Gain1/1
  [n_RPM_act] -> Gain2/1

== system New_FOC_old0x2820x29/FOC_SPWM/Decoupling//Coupling With Voltage Limits/MI_Calculations ==
  Vq_ref : Inport
  Vd_ref : Inport  Port=2
  Constant : Constant  Value=Vdc
  Divide : Product  Inputs=/*
  Gain7 : Gain  Gain=sqrt(3)
  Sqrt : Sqrt
  Square : Math  Operator=square
  Square1 : Math  Operator=square
  Sum4 : Sum  Inputs=|++
  MI : Outport
  wires:
  Sum4/1 -> Sqrt/1
  Square/1 -> Sum4/1
  Square1/1 -> Sum4/2
  Gain7/1 -> Divide/2
  [Vq_ref] -> Square/1
  Constant/1 -> Divide/1
  Sqrt/1 -> Gain7/1
  [Vd_ref] -> Square1/1
  Divide/1 -> MI/1
  Vq_ref/1 -> [Vq_ref]
  Vd_ref/1 -> [Vd_ref]

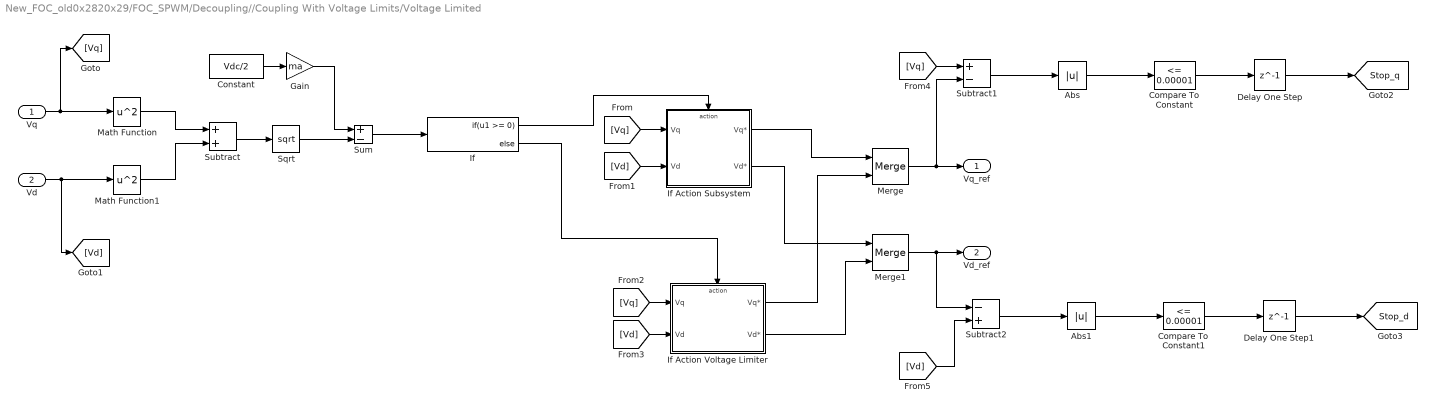
== system New_FOC_old0x2820x29/FOC_SPWM/Decoupling//Coupling With Voltage Limits/Voltage Limited ==
  Vq : Inport
  Vd : Inport  Port=2
  Abs : Abs  SaturateOnIntegerOverflow=off
  Abs1 : Abs  SaturateOnIntegerOverflow=off
  Compare To Constant : simulink/Logic and Bit Operations/Compare To Constant  relop=<=  const=0.00001  OutDataTypeStr=boolean
  Compare To Constant1 : simulink/Logic and Bit Operations/Compare To Constant  relop=<=  const=0.00001  OutDataTypeStr=boolean
  Constant : Constant  Value=Vdc/2
  Delay One Step : Delay  DelayLength=1
  Delay One Step1 : Delay  DelayLength=1
  Gain : Gain  Gain=ma
  If : If  IfExpression=u1 >= 0
  If Action Subsystem : Subsystem  TreatAsAtomicUnit=on
  If Action Voltage Limiter : Subsystem  TreatAsAtomicUnit=on
  Math Function : Math  Operator=square  SignedPower=on
  Math Function1 : Math  Operator=square  SignedPower=on
  Merge : Merge
  Merge1 : Merge
  Sqrt : Sqrt
  Subtract : Sum
  Subtract1 : Sum  Inputs=+-
  Subtract2 : Sum  Inputs=-+
  Sum : Sum  Inputs=+-
  Vq_ref : Outport
  Vd_ref : Outport  Port=2
  tag scope: Stop_d=global, Stop_q=global
  wires:
  [Vd] -> Subtract2/2
  Merge1/1 -> Vd_ref/1, Subtract2/1
  Subtract2/1 -> Abs1/1
  Abs1/1 -> Compare To Constant1/1
  Compare To Constant1/1 -> Delay One Step1/1
  Delay One Step1/1 -> [Stop_d]
  Delay One Step/1 -> [Stop_q]
  Compare To Constant/1 -> Delay One Step/1
  Abs/1 -> Compare To Constant/1
  Subtract1/1 -> Abs/1
  [Vq] -> Subtract1/1
  If Action Subsystem/2(Vd*) -> Merge1/1
  If Action Voltage Limiter/2(Vd*) -> Merge1/2
  If Action Voltage Limiter/1(Vq*) -> Merge/2
  If Action Subsystem/1(Vq*) -> Merge/1
  Merge/1 -> Vq_ref/1, Subtract1/2
  [Vd] -> If Action Voltage Limiter/2(Vd)
  [Vq] -> If Action Voltage Limiter/1(Vq)
  If/2 -> If Action Voltage Limiter/Action
  [Vd] -> If Action Subsystem/2(Vd)
  [Vq] -> If Action Subsystem/1(Vq)
  Vq/1 -> [Vq], Math Function/1
  If/1 -> If Action Subsystem/Action
  Gain/1 -> Sum/1
  Sum/1 -> If/1
  Constant/1 -> Gain/1
  Sqrt/1 -> Sum/2
  Subtract/1 -> Sqrt/1
  Math Function1/1 -> Subtract/2
  Math Function/1 -> Subtract/1
  Vd/1 -> Math Function1/1, [Vd]

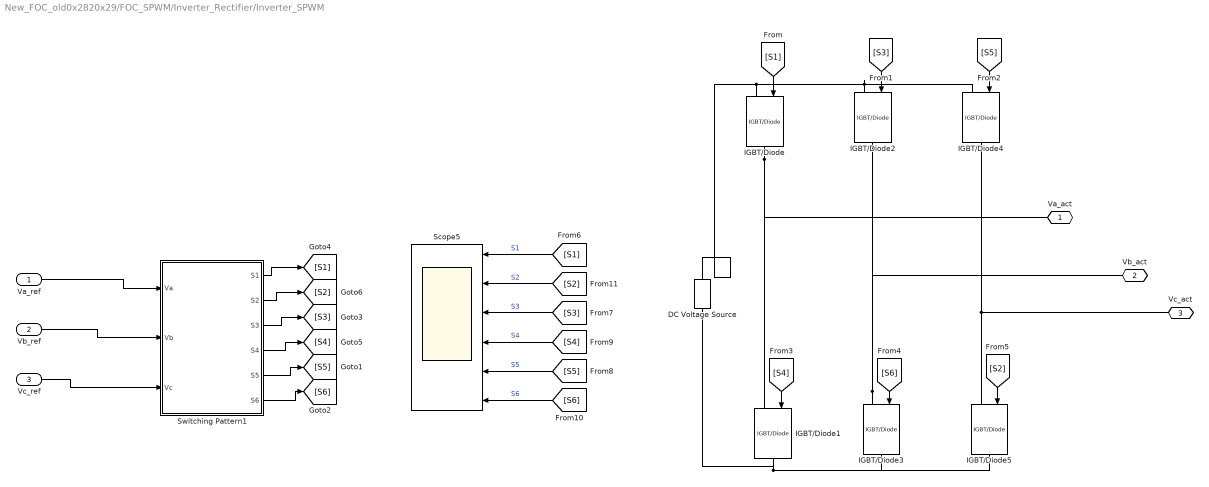
== system New_FOC_old0x2820x29/FOC_SPWM/Inverter_Rectifier/Inverter_SPWM ==
  Va_ref : Inport
  Vb_ref : Inport  Port=2
  Vc_ref : Inport  Port=3
  DC Voltage Source : spsDCVoltageSourceLib/DC Voltage Source  Amplitude=300  Measurements=None
  IGBT/Diode{,1..5} (6 alike) : spsIGBTDiodeLib/IGBT//Diode  Ron=1e-3  Rs=1e5  Cs=inf  Measurements=off
  Scope5 : Scope  NumInputPorts=6
  Switching Pattern1 : Subsystem
  Va_act : PMIOPort  Side=Right
  Vb_act : PMIOPort  Port=2  Side=Right
  Vc_act : PMIOPort  Port=3  Side=Right
  wires:
  Switching Pattern1/1(S1) -> [S1]
  Switching Pattern1/2(S2) -> [S2]
  Switching Pattern1/3(S3) -> [S3]
  Switching Pattern1/6(S6) -> [S6]
  Va_ref/1 -> Switching Pattern1/1(Va)
  Switching Pattern1/5(S5) -> [S5]
  Vb_ref/1 -> Switching Pattern1/2(Vb)
  Vc_ref/1 -> Switching Pattern1/3(Vc)
  Switching Pattern1/4(S4) -> [S4]
  [S5] -> IGBT/Diode4/1
  [S2] -> Scope5/2  "S2"
  [S5] -> Scope5/5  "S5"
  [S6] -> Scope5/6  "S6"
  [S2] -> IGBT/Diode5/1
  [S4] -> IGBT/Diode1/1
  [S1] -> IGBT/Diode/1
  [S1] -> Scope5/1  "S1"
  [S6] -> IGBT/Diode3/1
  [S3] -> Scope5/3  "S3"
  [S3] -> IGBT/Diode2/1
  [S4] -> Scope5/4  "S4"
  connections:
  Vc_act/RConn1 -- IGBT/Diode5/LConn1 -- IGBT/Diode4/RConn1
  IGBT/Diode2/LConn1 -- DC Voltage Source/RConn1 -- IGBT/Diode/LConn1 -- IGBT/Diode4/LConn1
  IGBT/Diode1/RConn1 -- DC Voltage Source/LConn1 -- IGBT/Diode3/RConn1 -- IGBT/Diode5/RConn1
  IGBT/Diode3/LConn1 -- Vb_act/RConn1 -- IGBT/Diode2/RConn1
  IGBT/Diode/RConn1 -- Va_act/RConn1 -- IGBT/Diode1/LConn1

== system New_FOC_old0x2820x29/FOC_SVPWM/Decoupling//Coupling With Voltage Limits/Decoupling//Coupling ==
  Vq_hat : Inport
  Vd_hat : Inport  Port=2
  Constant1 : Constant  Value=lambda
  Constant3 : Constant  Value=Ld
  Constant5 : Constant  Value=Lq
  Product3 : Product
  Product4 : Product  Inputs=3
  Product5 : Product  Inputs=3
  Sum1 : Sum  Inputs=|+-
  Sum2 : Sum  Inputs=+++
  Vq : Outport
  Vd : Outport  Port=2
  wires:
  [Wm_actual] -> Product4/1
  [Wm_actual] -> Product3/1
  Constant3/1 -> Product4/2
  Constant5/1 -> Product5/2
  [Id_actual] -> Product4/3
  Vd_hat/1 -> Sum1/1
  Constant1/1 -> Product3/2
  [Wm_actual] -> Product5/1
  [Iq_actual] -> Product5/3
  Product4/1 -> Sum2/1
  Vq_hat/1 -> Sum2/2
  Product3/1 -> Sum2/3
  Product5/1 -> Sum1/2
  Sum2/1 -> Vq/1
  Sum1/1 -> Vd/1

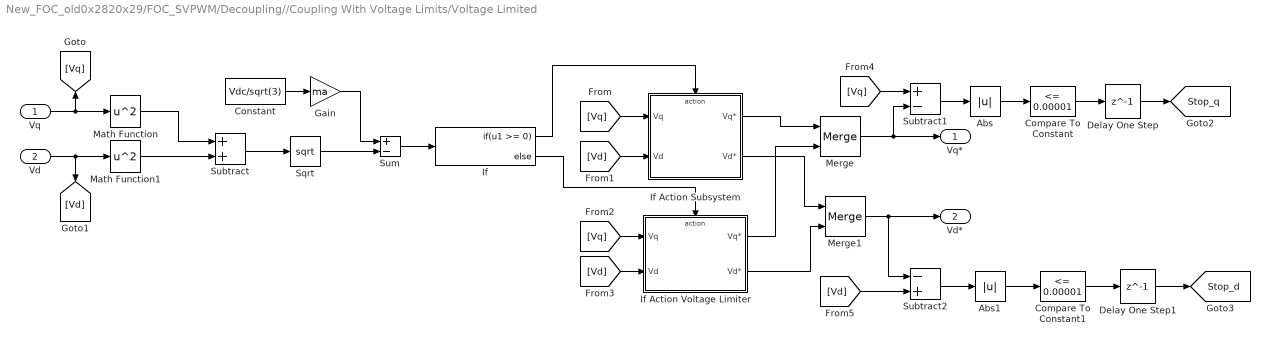
== system New_FOC_old0x2820x29/FOC_SVPWM/Decoupling//Coupling With Voltage Limits/Voltage Limited ==
  Vq : Inport
  Vd : Inport  Port=2
  Abs : Abs  SaturateOnIntegerOverflow=off
  Abs1 : Abs  SaturateOnIntegerOverflow=off
  Compare To Constant : simulink/Logic and Bit Operations/Compare To Constant  relop=<=  const=0.00001  OutDataTypeStr=boolean
  Compare To Constant1 : simulink/Logic and Bit Operations/Compare To Constant  relop=<=  const=0.00001  OutDataTypeStr=boolean
  Constant : Constant  Value=Vdc/sqrt(3)
  Delay One Step : Delay  DelayLength=1
  Delay One Step1 : Delay  DelayLength=1
  Gain : Gain  Gain=ma
  If : If  IfExpression=u1 >= 0
  If Action Subsystem : Subsystem  TreatAsAtomicUnit=on
  If Action Voltage Limiter : Subsystem  TreatAsAtomicUnit=on
  Math Function : Math  Operator=square  SignedPower=on
  Math Function1 : Math  Operator=square  SignedPower=on
  Merge : Merge
  Merge1 : Merge
  Sqrt : Sqrt
  Subtract : Sum
  Subtract1 : Sum  Inputs=+-
  Subtract2 : Sum  Inputs=-+
  Sum : Sum  Inputs=+-
  Vq* : Outport
  Vd* : Outport  Port=2
  tag scope: Stop_d=global, Stop_q=global
  wires:
  Vd/1 -> [Vd], Math Function1/1
  Math Function/1 -> Subtract/1
  Math Function1/1 -> Subtract/2
  Subtract/1 -> Sqrt/1
  Sqrt/1 -> Sum/2
  Constant/1 -> Gain/1
  Sum/1 -> If/1
  Gain/1 -> Sum/1
  If/1 -> If Action Subsystem/Action
  Vq/1 -> Math Function/1, [Vq]
  [Vq] -> If Action Subsystem/1(Vq)
  [Vd] -> If Action Subsystem/2(Vd)
  If/2 -> If Action Voltage Limiter/Action
  [Vq] -> If Action Voltage Limiter/1(Vq)
  [Vd] -> If Action Voltage Limiter/2(Vd)
  Merge/1 -> Vq*/1, Subtract1/2
  If Action Subsystem/1(Vq*) -> Merge/1
  If Action Voltage Limiter/1(Vq*) -> Merge/2
  If Action Voltage Limiter/2(Vd*) -> Merge1/2
  If Action Subsystem/2(Vd*) -> Merge1/1
  [Vq] -> Subtract1/1
  Subtract1/1 -> Abs/1
  Abs/1 -> Compare To Constant/1
  Compare To Constant/1 -> Delay One Step/1
  Delay One Step/1 -> [Stop_q]
  Delay One Step1/1 -> [Stop_d]
  Compare To Constant1/1 -> Delay One Step1/1
  Abs1/1 -> Compare To Constant1/1
  Subtract2/1 -> Abs1/1
  Merge1/1 -> Vd*/1, Subtract2/1
  [Vd] -> Subtract2/2

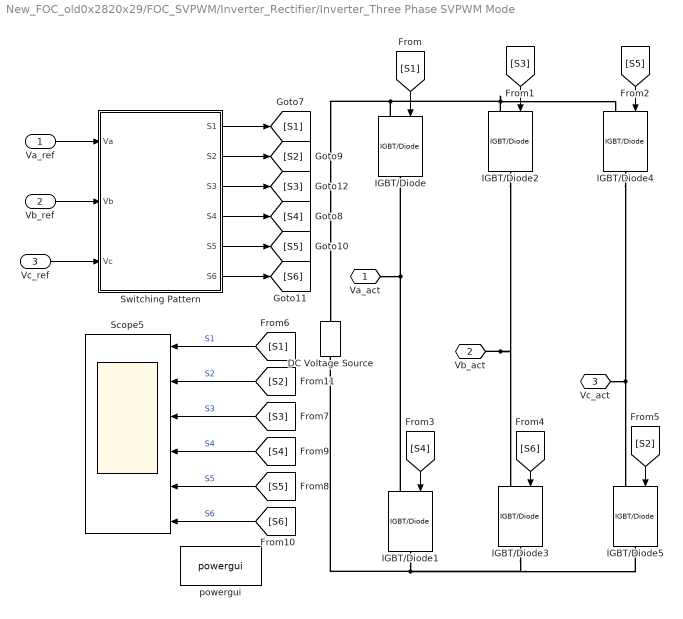
== system New_FOC_old0x2820x29/FOC_SVPWM/Inverter_Rectifier/Inverter_Three Phase SVPWM Mode ==
  Va_ref : Inport
  Vb_ref : Inport  Port=2
  Vc_ref : Inport  Port=3
  DC Voltage Source : spsDCVoltageSourceLib/DC Voltage Source  Amplitude=Vdc  Measurements=None
  IGBT/Diode{,1..5} (6 alike) : spsIGBTDiodeLib/IGBT//Diode  Ron=1e-3  Rs=1e5  Cs=inf  Measurements=off
  Scope5 : Scope  NumInputPorts=6
  Switching Pattern : Subsystem
  powergui : spspowerguiLib/powergui  Priority=1  SimulationMode=Continuous  SampleTime=50e-6  frequency=60  Iterations=50  frequencyindice=0  Pbase=100e6  ErrMax=1e-4  UnitsV=kV  UnitsW=MW  buscounter=0  FunctionMessages=off  echomessages=off  EnableUseOfTLC=off  CurrentSourceSwitches=off  DisableSnubberDevices=off  DisableRonSwitches=off  DisableVfSwitches=off  DisplayEquations=off  AutomaticDiscreteSolvers=off  SolverType=Tustin/Backward Euler (TBE)  Interpol=off  ExternalGateDelay=off  methode=off  Ts=100  x0status=blocks  SPID=on  SwTol=0  HookPort=off  NonlinearTolerance=1e-4  nMaxIteration=100  ContinueOnMaxIteration=off  RestoreLinks=warning  ResistiveCurrentMeasurement=off  Frange=[0:2:500]  Ylog=off  Xlog=on  ShowGrid=off  save=off  variable=ZData  structure=0  ZoomFFT=off  StartTime=0.0  cycles=1  DisplayStyle=1  fundamental=60  FreqAxis=off  MaxFrequency=1000  frequencyindicesteady=1  RmsSteady=1  display=off
  Va_act : PMIOPort  Side=Right
  Vb_act : PMIOPort  Port=2  Side=Right
  Vc_act : PMIOPort  Port=3  Side=Right
  wires:
  Vc_ref/1 -> Switching Pattern/3(Vc)
  Vb_ref/1 -> Switching Pattern/2(Vb)
  Va_ref/1 -> Switching Pattern/1(Va)
  [S5] -> IGBT/Diode4/1
  [S2] -> Scope5/2  "S2"
  [S5] -> Scope5/5  "S5"
  Switching Pattern/4(S4) -> [S4]
  Switching Pattern/3(S3) -> [S3]
  [S6] -> Scope5/6  "S6"
  [S2] -> IGBT/Diode5/1
  [S4] -> IGBT/Diode1/1
  [S1] -> IGBT/Diode/1
  Switching Pattern/2(S2) -> [S2]
  [S1] -> Scope5/1  "S1"
  [S6] -> IGBT/Diode3/1
  [S3] -> Scope5/3  "S3"
  [S3] -> IGBT/Diode2/1
  Switching Pattern/1(S1) -> [S1]
  Switching Pattern/6(S6) -> [S6]
  Switching Pattern/5(S5) -> [S5]
  [S4] -> Scope5/4  "S4"
  connections:
  Vc_act/RConn1 -- IGBT/Diode4/RConn1 -- IGBT/Diode5/LConn1
  IGBT/Diode2/LConn1 -- DC Voltage Source/RConn1 -- IGBT/Diode/LConn1 -- IGBT/Diode4/LConn1
  IGBT/Diode1/RConn1 -- IGBT/Diode3/RConn1 -- IGBT/Diode5/RConn1 -- DC Voltage Source/LConn1
  Vb_act/RConn1 -- IGBT/Diode3/LConn1 -- IGBT/Diode2/RConn1
  Va_act/RConn1 -- IGBT/Diode/RConn1 -- IGBT/Diode1/LConn1

== system New_FOC_old0x2820x29/FOC_SPWM/Decoupling//Coupling With Voltage Limits/Voltage Limited/If Action Subsystem ==
  Vq : Inport
  Vd : Inport  Port=2
  Action Port : ActionPort  ActionPortLabel=if(u1 >= 0)
  Data Type Conversion : DataTypeConversion  OutDataTypeStr=double  SaturateOnIntegerOverflow=off  RndMeth=Floor
  Data Type Conversion1 : DataTypeConversion  OutDataTypeStr=double  SaturateOnIntegerOverflow=off  RndMeth=Floor
  Vq* : Outport
  Vd* : Outport  Port=2
  wires:
  Vd/1 -> Data Type Conversion1/1
  Vq/1 -> Data Type Conversion/1
  Data Type Conversion/1 -> Vq*/1
  Data Type Conversion1/1 -> Vd*/1

== system New_FOC_old0x2820x29/FOC_SPWM/Decoupling//Coupling With Voltage Limits/Voltage Limited/If Action Voltage Limiter ==
  Vq : Inport
  Vd : Inport  Port=2
  Action Port : ActionPort  ActionPortLabel=else
  Divide : Product  Inputs=*/
  Divide1 : Product  Inputs=/*
  Gain : Gain  Gain=Vdc*ma
  Gain1 : Gain  Gain=2
  Gain2 : Gain  Gain=Vdc*ma
  Math Function : Math  Operator=square  SignedPower=on
  Math Function1 : Math  Operator=square  SignedPower=on
  Sqrt : Sqrt
  Subtract : Sum
  Vq* : Outport
  Vd* : Outport  Port=2
  wires:
  Divide1/1 -> Vd*/1
  Divide/1 -> Vq*/1
  Gain2/1 -> Divide1/2
  Gain1/1 -> Divide/2, Divide1/1
  Vd/1 -> Math Function1/1, Gain2/1
  Math Function1/1 -> Subtract/2
  Gain/1 -> Divide/1
  Vq/1 -> Math Function/1, Gain/1
  Math Function/1 -> Subtract/1
  Sqrt/1 -> Gain1/1
  Subtract/1 -> Sqrt/1

== system New_FOC_old0x2820x29/FOC_SPWM/Inverter_Rectifier/Inverter_SPWM/Switching Pattern1 ==
  Va : Inport
  Vb : Inport  Port=2
  Vc : Inport  Port=3
  Gain : Gain  Gain=2/Vdc
  Gain1 : Gain  Gain=2/Vdc
  Gain2 : Gain  Gain=2/Vdc
  NOT3 : Logic  Operator=NOT  IconShape=distinctive  AllPortsSameDT=off  OutDataTypeStr=boolean
  NOT4 : Logic  Operator=NOT  IconShape=distinctive  AllPortsSameDT=off  OutDataTypeStr=boolean
  NOT5 : Logic  Operator=NOT  IconShape=distinctive  AllPortsSameDT=off  OutDataTypeStr=boolean
  Relational Operator : RelationalOperator  Operator=>  OutDataTypeStr=boolean  ZeroCross=off  RndMeth=Simplest  InputSameDT=off
  Relational Operator1 : RelationalOperator  Operator=>  OutDataTypeStr=boolean  ZeroCross=off  RndMeth=Simplest  InputSameDT=off
  Relational Operator2 : RelationalOperator  Operator=>  OutDataTypeStr=boolean  ZeroCross=off  RndMeth=Simplest  InputSameDT=off
  Scope : Scope  NumInputPorts=4
  Scope1 : Scope  NumInputPorts=4
  Triangle Generator1 : spsTriangleGeneratorLib/Triangle Generator  Freq=fs  Phase=90  Ts=0
  S1 : Outport
  S2 : Outport  Port=2
  S3 : Outport  Port=3
  S4 : Outport  Port=4
  S5 : Outport  Port=5
  S6 : Outport  Port=6
  wires:
  Triangle Generator1/1 -> Scope1/4, Scope/4, Relational Operator/2, Relational Operator1/2, Relational Operator2/2
  NOT5/1 -> S2/1
  Relational Operator2/1 -> NOT5/1, S5/1
  NOT4/1 -> S6/1
  Relational Operator1/1 -> NOT4/1, S3/1
  NOT3/1 -> S4/1
  [vb] -> Relational Operator1/1
  [vc] -> Relational Operator2/1
  [va] -> Relational Operator/1
  Va/1 -> Scope/1, Gain/1
  Vb/1 -> Scope/2, Gain1/1
  Vc/1 -> Scope/3, Gain2/1
  Relational Operator/1 -> NOT3/1, S1/1
  Gain/1 -> Scope1/1, [va]
  Gain1/1 -> Scope1/2, [vb]
  Gain2/1 -> Scope1/3, [vc]

== system New_FOC_old0x2820x29/FOC_SVPWM/Decoupling//Coupling With Voltage Limits/Voltage Limited/If Action Subsystem ==
  Vq : Inport
  Vd : Inport  Port=2
  Action Port : ActionPort  ActionPortLabel=if(u1 >= 0)
  Data Type Conversion : DataTypeConversion  OutDataTypeStr=double  SaturateOnIntegerOverflow=off  RndMeth=Floor
  Data Type Conversion1 : DataTypeConversion  OutDataTypeStr=double  SaturateOnIntegerOverflow=off  RndMeth=Floor
  Vq* : Outport
  Vd* : Outport  Port=2
  wires:
  Data Type Conversion1/1 -> Vd*/1
  Data Type Conversion/1 -> Vq*/1
  Vq/1 -> Data Type Conversion/1
  Vd/1 -> Data Type Conversion1/1

== system New_FOC_old0x2820x29/FOC_SVPWM/Decoupling//Coupling With Voltage Limits/Voltage Limited/If Action Voltage Limiter ==
  Vq : Inport
  Vd : Inport  Port=2
  Action Port : ActionPort  ActionPortLabel=else
  Divide : Product  Inputs=*/
  Divide1 : Product  Inputs=/*
  Gain : Gain  Gain=Vdc*ma
  Gain1 : Gain  Gain=sqrt(3)
  Gain2 : Gain  Gain=Vdc*ma
  Math Function : Math  Operator=square  SignedPower=on
  Math Function1 : Math  Operator=square  SignedPower=on
  Sqrt : Sqrt
  Subtract : Sum
  Vq* : Outport
  Vd* : Outport  Port=2
  wires:
  Subtract/1 -> Sqrt/1
  Vq/1 -> Gain/1, Math Function/1
  Vd/1 -> Gain2/1, Math Function1/1
  Math Function/1 -> Subtract/1
  Gain2/1 -> Divide1/2
  Math Function1/1 -> Subtract/2
  Gain/1 -> Divide/1
  Sqrt/1 -> Gain1/1
  Gain1/1 -> Divide1/1, Divide/2
  Divide/1 -> Vq*/1
  Divide1/1 -> Vd*/1

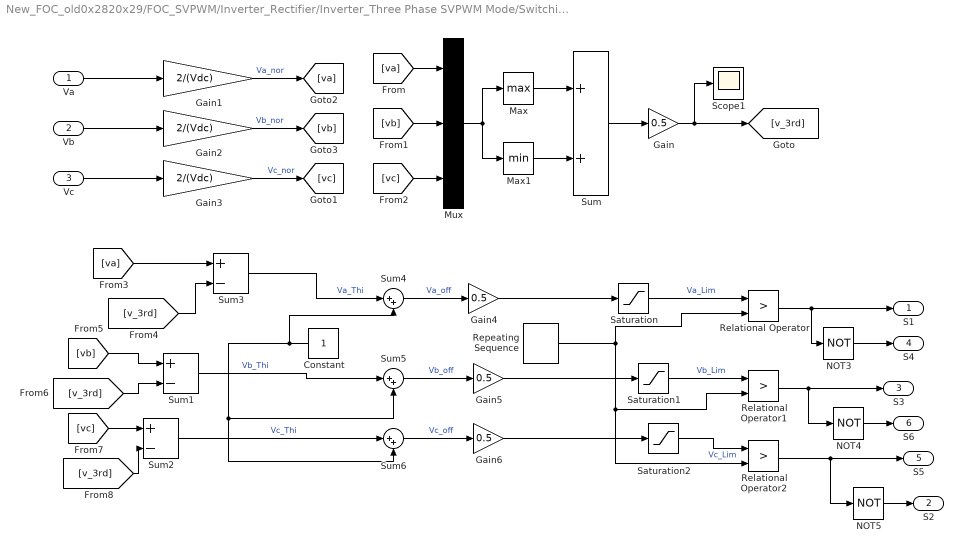
== system New_FOC_old0x2820x29/FOC_SVPWM/Inverter_Rectifier/Inverter_Three Phase SVPWM Mode/Switching Pattern ==
  Va : Inport
  Vb : Inport  Port=2
  Vc : Inport  Port=3
  Constant : Constant
  Gain{,4..6} (4 alike) : Gain  Gain=0.5
  Gain1 : Gain  Gain=2/(Vdc)  ParamDataTypeStr=single  OutDataTypeStr=single
  Gain2 : Gain  Gain=2/(Vdc)  ParamDataTypeStr=single  OutDataTypeStr=single
  Gain3 : Gain  Gain=2/(Vdc)  ParamDataTypeStr=single  OutDataTypeStr=single
  Max : MinMax  Function=max
  Max1 : MinMax
  Mux : Mux  Inputs=3
  NOT3 : Logic  Operator=NOT  IconShape=distinctive  AllPortsSameDT=off  OutDataTypeStr=boolean
  NOT4 : Logic  Operator=NOT  IconShape=distinctive  AllPortsSameDT=off  OutDataTypeStr=boolean
  NOT5 : Logic  Operator=NOT  IconShape=distinctive  AllPortsSameDT=off  OutDataTypeStr=boolean
  Relational Operator : RelationalOperator  Operator=>  OutDataTypeStr=boolean  RndMeth=Simplest  InputSameDT=off
  Relational Operator1 : RelationalOperator  Operator=>  OutDataTypeStr=boolean  RndMeth=Simplest  InputSameDT=off
  Relational Operator2 : RelationalOperator  Operator=>  OutDataTypeStr=boolean  RndMeth=Simplest  InputSameDT=off
  Repeating Sequence : simulink/Sources/Repeating Sequence  rep_seq_t=[ 0 (T_period)/2 (T_period) ]  rep_seq_y=[ 0 (1) 0 ]
  Saturation : Saturate  UpperLimit=1  LowerLimit=0  LinearizeAsGain=off  ZeroCross=off
  Saturation1 : Saturate  UpperLimit=1  LowerLimit=0  LinearizeAsGain=off  ZeroCross=off
  Saturation2 : Saturate  UpperLimit=1  LowerLimit=0  LinearizeAsGain=off  ZeroCross=off
  Scope1 : Scope
  Sum : Sum
  Sum1 : Sum  Inputs=+-
  Sum2 : Sum  Inputs=+-
  Sum3 : Sum  Inputs=+-
  Sum4 : Sum  Inputs=|++
  Sum5 : Sum  Inputs=|++
  Sum6 : Sum  Inputs=|++
  S1 : Outport
  S2 : Outport  Port=2
  S3 : Outport  Port=3
  S4 : Outport  Port=4
  S5 : Outport  Port=5
  S6 : Outport  Port=6
  wires:
  Vc/1 -> Gain3/1
  Vb/1 -> Gain2/1
  Va/1 -> Gain1/1
  [vc] -> Mux/3
  [vb] -> Mux/2
  [va] -> Mux/1
  Repeating Sequence/1 -> Relational Operator2/2, Relational Operator1/2, Relational Operator/2
  Gain/1 -> [v_3rd], Scope1/1
  [va] -> Sum3/1
  Mux/1 -> Max1/1, Max/1
  [vc] -> Sum2/1
  [vb] -> Sum1/1
  Sum/1 -> Gain/1
  [v_3rd] -> Sum3/2
  [v_3rd] -> Sum2/2
  [v_3rd] -> Sum1/2
  Max/1 -> Sum/1
  Max1/1 -> Sum/2
  Relational Operator/1 -> S1/1, NOT3/1
  NOT3/1 -> S4/1
  Relational Operator1/1 -> NOT4/1, S3/1
  NOT4/1 -> S6/1
  Relational Operator2/1 -> NOT5/1, S5/1
  NOT5/1 -> S2/1
  Saturation/1 -> Relational Operator/1  "Va_Lim"
  Saturation1/1 -> Relational Operator1/1  "Vb_Lim"
  Saturation2/1 -> Relational Operator2/1  "Vc_Lim"
  Gain1/1 -> [va]  "Va_nor"
  Gain2/1 -> [vb]  "Vb_nor"
  Gain3/1 -> [vc]  "Vc_nor"
  Sum1/1 -> Sum5/1  "Vb_Thi"
  Sum5/1 -> Gain5/1  "Vb_off"
  Sum2/1 -> Sum6/1  "Vc_Thi"
  Sum6/1 -> Gain6/1  "Vc_off"
  Constant/1 -> Sum6/2, Sum5/2, Sum4/2
  Gain5/1 -> Saturation1/1
  Gain6/1 -> Saturation2/1
  Sum4/1 -> Gain4/1  "Va_off"
  Gain4/1 -> Saturation/1
  Sum3/1 -> Sum4/1  "Va_Thi"
